simulink model "z4_1"  (R2017b)
settings: Solver=FixedStepDiscrete  StartTime=0.0  StopTime=0  RelTol=1e-3
undefined symbols (not defined in the file or in its folder): W
libraries: CPOiS_SourcesSinks x7, CPOiS_LinearTransforms x2, CPOiS_Filters x1, CPOiS_DataManipulation_DataTypeConversion x1
settings Model: Creator=alis  LastModifiedBy=alis

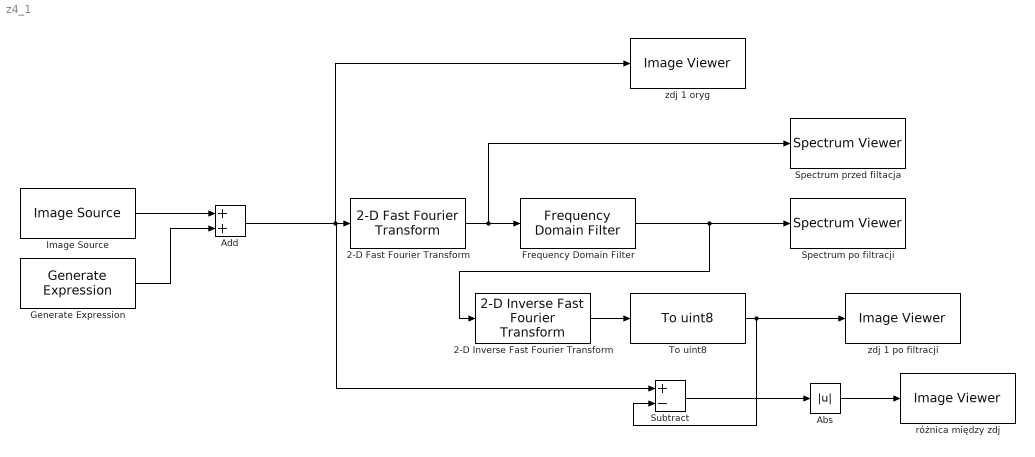
== system z4_1 ==
  2-D Fast Fourier Transform : CPOiS_LinearTransforms/2-D Fast Fourier Transform
      settings: SourceProductName=CPOiS - Digital image and signal processing
  2-D Inverse Fast Fourier Transform : CPOiS_LinearTransforms/2-D Inverse Fast  Fourier Transform
      settings: SourceProductName=CPOiS - Digital image and signal processing
  Abs : Abs
  Add : Sum
  Frequency Domain Filter : CPOiS_Filters/Frequency Domain Filter  filtertype=Low-pass Filter  radius=50
      settings: SourceProductName=CPOiS - Digital image and signal processing
  Generate Expression : CPOiS_SourcesSinks/Generate Expression  Width=512  Height=512  Expression=128.*(sin(W)+1)
      settings: SourceProductName=CPOiS - Digital image and signal processing
  Image Source : CPOiS_SourcesSinks/Image Source  FileSelection=ball.png
      settings: SourceProductName=CPOiS - Digital image and signal processing
  Spectrum po filtracji : CPOiS_SourcesSinks/Spectrum Viewer
      settings: SourceProductName=CPOiS - Digital image and signal processing
  Spectrum przed filtacja : CPOiS_SourcesSinks/Spectrum Viewer
      settings: SourceProductName=CPOiS - Digital image and signal processing
  Subtract : Sum  Inputs=+-
  To uint8 : CPOiS_DataManipulation_DataTypeConversion/To uint8
      settings: SourceProductName=CPOiS - Digital image and signal processing
  "różnica między zdj " : CPOiS_SourcesSinks/Image Viewer
      settings: SourceProductName=CPOiS - Digital image and signal processing
  zdj 1 oryg : CPOiS_SourcesSinks/Image Viewer
      settings: SourceProductName=CPOiS - Digital image and signal processing
  zdj 1 po filtracji : CPOiS_SourcesSinks/Image Viewer
      settings: SourceProductName=CPOiS - Digital image and signal processing
  wires:
  2-D Fast Fourier Transform/1 -> Spectrum przed filtacja/1, Frequency Domain Filter/1
  Image Source/1 -> Add/1
  Abs/1 -> "różnica między zdj "/1
  Subtract/1 -> Abs/1
  2-D Inverse Fast Fourier Transform/1 -> To uint8/1
  Frequency Domain Filter/1 -> 2-D Inverse Fast Fourier Transform/1, Spectrum po filtracji/1
  To uint8/1 -> Subtract/2, zdj 1 po filtracji/1
  Add/1 -> Subtract/1, zdj 1 oryg/1, 2-D Fast Fourier Transform/1
  Generate Expression/1 -> Add/2
